simulink model "Yes"  (R2018b)
settings: Solver=VariableStepAuto  StartTime=0.0  StopTime=1  RelTol=1e-3
settings Model: Creator=kekos  LastModifiedBy=kekos

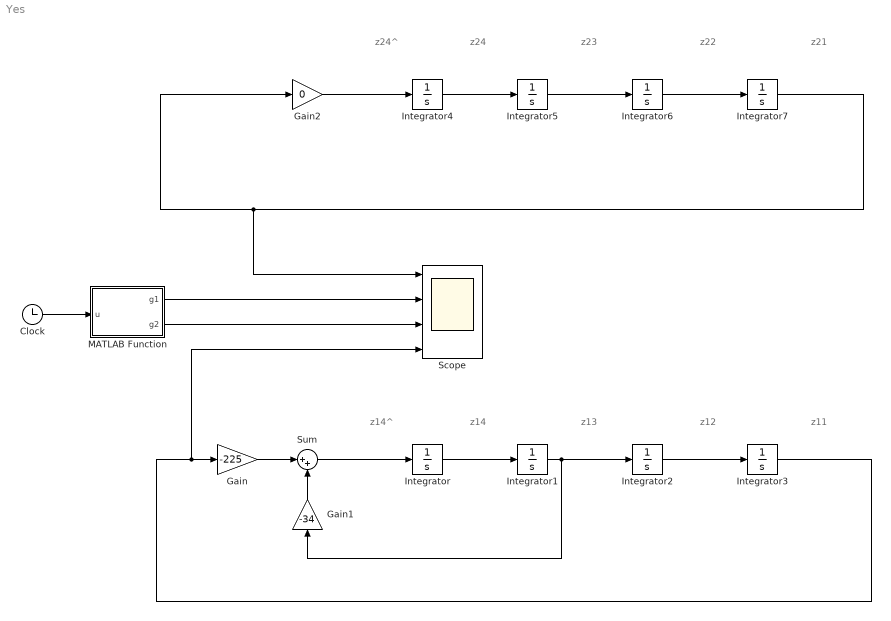
== system Yes ==
  note: z11
  note: z12
  note: z13
  note: z14
  note: z14^
  note: z24^
  note: z24
  note: z23
  note: z22
  note: z21
  Clock : Clock
  Gain : Gain  Gain=-225
  Gain1 : Gain  Gain=-34
  Gain2 : Gain  Gain=0
  Integrator : Integrator  InitialCondition=-49
  Integrator{1,3..4,6..7} (5 alike) : Integrator
  Integrator2 : Integrator  InitialCondition=1
  Integrator5 : Integrator  InitialCondition=2
  MATLAB Function : MATLAB Function  TreatAsAtomicUnit=on
  Scope : Scope  NumInputPorts=4
  Sum : Sum  Inputs=|++
  wires:
  Clock/1 -> MATLAB Function/1(u)
  Integrator/1 -> Integrator1/1
  Integrator1/1 -> Integrator2/1, Gain1/1
  Integrator2/1 -> Integrator3/1
  Integrator3/1 -> Scope/4, Gain/1
  Gain1/1 -> Sum/2
  Gain/1 -> Sum/1
  Sum/1 -> Integrator/1
  Integrator7/1 -> Scope/1, Gain2/1
  Gain2/1 -> Integrator4/1
  Integrator4/1 -> Integrator5/1
  Integrator5/1 -> Integrator6/1
  Integrator6/1 -> Integrator7/1
  MATLAB Function/1(g1) -> Scope/2
  MATLAB Function/2(g2) -> Scope/3

== matlab function Yes/MATLAB Function ==
  data: u input; g1 output; g2 output
function [g1,g2] = fcn(u)

g2 = sin(u)*cos(4*u);
g1 = u^2;
